simulink model "TestonBESSPVPlant"  (R2026a)
settings: Solver=VariableStepAuto  StopTime=SimulationTime  FixedStep=Ts
PreLoadFcn:
  | testModelparameters;
undefined symbols (not defined in the file): Array, Base, battery, BatteryInverter, DiscIntNeverNeededParam, fRT, GFLBatteryController, GFMBatteryController, Grid, LVRT, Panel, PVController, PVInverter, Qtrack, Ts, VSMbase
libraries: nesl_utility x16, eeGeneralControl x15, ee_lib x10, simulink x7, eeTransforms x6, fl_lib x5, eePowerMeasurement x5, slpidlib x2, batteryecm_lib x1, simulink_extras x1
(part 2 of 3)

== system TestonBESSPVPlant/BESS PV PARK/60 MWhr Battery Energy Storage/Variant Subsystem/Grid Forming VSM ==
  In Bus Element : Inport  PortName=Bat  Element=Iabc_bat
  In Bus Element1 : Inport  PortName=Bat  Element=Vabc_bat
  Constant : Constant  Value=GFMBatteryController.P_ref*0 +0.3  SampleTime=Ts
  Constant1 : Constant  Value=GFMBatteryController.Q_ref*0+0.01  SampleTime=Ts
  From Workspace : FromWorkspace  VariableName=reference.Flat  SampleTime=Ts
  From Workspace1 : FromWorkspace  VariableName=reference.Flat  SampleTime=Ts
  GridFormingController : Subsystem  mask(Grid-Forming Controller){power=VSMbase.power*1e3, girdLineVoltage=VSMbase.lineVoltage, powerFreq=VSMbase.frequency, dcBusVoltage=BatteryInverter.DCVoltage, measSampleTime=GFMBatteryController.Sampletime, powerControl=Virtual Synchronous Machine, activePowerSampleTime=GFMBatteryController.Sampletime, droopSlope=BatteryInverter.droopControl.freqSlopeMp, droopT1=BatteryInverter.droopControl.T1, droopT2=BatteryInverter.droopControl.T2, droopTC=BatteryInverter.droopControl.lpfTimeConst, vsmPmeasFilterTC=GFMBatteryController.filtertimeconstant, vsmFreqDroop=1/GFMBatteryController.frequencydroop, vsmInertiaTC=GFMBatteryController.VSMInertia, vsmDampingConst=GFMBatteryController.Damping, dampingPowerMaxLimit=1, dampingPowerMinLimit=-1, freqMeasTimeConst=GFMBatteryController.frequencymeastimeconstant, freqOption=Grid Frequency Measurement, voltreference=GFMBatteryController.voltagref, QVoltFilterTC=GFMBatteryController.reactivepowerfiltertimeconstant, QVoltDroop=GFMBatteryController.voltagedroop, lowVoltageSupportGain=GFMBatteryController.voltagsupportgain, currentLimit=Virtual Impedance and Current Limiting, maxSatCurrentLimit=BatteryInverter.currentLimit.overNominalCurrent, maxVICurrentLimit=GFMBatteryController.maximumvirtualimpedancecurrent, ctLimitVirtualImp=BatteryInverter.currentLimit.virImpResistance, ctLimitXbyR=BatteryInverter.currentLimit.virImpXbyR, ctLimitDelayTime=10*GFMBatteryController.Sampletime, currentSatTime=0.001, currentVITimeConst=GFMBatteryController.virtimeconstant, modeTransferTime=0.01, voltControlTs=GFMBatteryController.voltagecontroltimeconstant, vdPGain=GFMBatteryController.voltagecontrolkp, VdIGain=GFMBatteryController.voltagecontrolki, VdMaxCt=1.8, VdMinCt=-1.8, VqPGain=GFMBatteryController.voltagecontrolkp, VqIGain=GFMBatteryController.voltagecontrolki, VqMaxCt=1.8, VqMinCt=-1.8, vdvqLPFTimeConst=GFMBatteryController.voltagecontroltimeconstant, currentControlTs=GFMBatteryController.currentcontrollersampletime, filterInductance=BatteryInverter.L, IdPGain=GFMBatteryController.currentcontrollerkp, IdIGain=GFMBatteryController.currentcontrollerki, IqPGain=GFMBatteryController.currentcontrollerkp, IqIGain=GFMBatteryController.currentcontrollerki}
      mask prompts: power "Grid-forming converter power (VA)"; girdLineVoltage "Grid line voltage (V)"; powerFreq "Grid frequency (Hz)"; dcBusVoltage "DC bus voltage (V)"; measSampleTime "Measurement sample time (s)"; powerControl "Active Power Control"; activePowerSampleTime "Power controller sample time (s)"; droopSlope "Power droop slope (pu, Hz/W)"; droopT1 "Lead-Lag numerator time constant (s)"; droopT2 "Lead-Lag denominator time constant (s)"; droopTC "Filter cut-off time constant (s)"; vsmPmeasFilterTC "Power measurement filter time constant (s)"; vsmFreqDroop "Frequency droop (pu,  W/Hz)"; vsmInertiaTC "Inertia constant M (pu)"; vsmDampingConst "Damping constant (pu/Hz)"; dampingPowerMaxLimit "Damping power maximum limit (pu)"; dampingPowerMinLimit "Damping power minimum limit (pu)"; freqMeasTimeConst "Frequency measurement time constant (s)"; freqOption "Damping power frequency option"; voltreference "Voltage reference value (pu)"; QVoltFilterTC "Power measurement filter time constant (s)"; QVoltDroop "Voltage droop (pu, V/VAr)"; lowVoltageSupportGain "Low voltage support gain (pu, A/V)"; currentLimit "Current limiting method"; maxSatCurrentLimit "Maximum current saturation (pu)"; maxVICurrentLimit "Maximum virtual impedance current (pu)"; ctLimitVirtualImp "Virtual impedance coefficient (pu.Ohm/pu.A)"; ctLimitXbyR "Virtual X/R ratio"; ctLimitDelayTime "Maximum current delay time (s)"; currentSatTime "Current limiting run time (s)"; currentVITimeConst "Filter time constant (s)"; modeTransferTime "Mode transfer time (s)"; voltControlTs "Voltage controller sample time (s)"; vdPGain "Vd proportional gain"; VdIGain "Vd integral gain"; VdMaxCt "Vd maximum current limit (A)"; VdMinCt "Vd minimum current limit (A)"; VqPGain "Vq proportional gain"; VqIGain "Vq integral gain"; VqMaxCt "Vq maximum current limit (A)"; VqMinCt "Vq minimum current limit (A)"; vdvqLPFTimeConst "Voltage measurement filter time constant (s)"; currentControlTs "Current controller sample time (s)"; filterInductance "Filter inductance (H)"; IdPGain "Id proportional gain"; IdIGain "Id integral gain"; IqPGain "Iq proportional gain"; IqIGain "Iq integral gain"
      mask help: This block implements the grid forming controller with fault ride through capability. Input to the controller are active and reactive power reference in per unit and the sensed three-phase phase current in amphere and phase voltage in volts.
      mask init:
      | powerChoice = get_param(gcb,'powerControl');
      | currentChoice = get_param(gcb,'currentLimit');
      | 
      | powerloc = [gcb, '/Power Control/ActivePowerControl']; 
      | currentloc = [gcb, '/Current Limiting/CurrentLimitingMethod'];
      | freqLoc = [gcb,'/Power Control/ActivePowerControl/vsmControl/Damping Frequency'];
      | 
      | switch powerChoice
      |     case 'Virtual Synchronous Machine'
      |         set_param(powerloc, 'LabelModeActiveChoice', 'vsm');
      |         dampingFreqChoice = get_param(gcb,'freqOption');
      |         if strcmp(dampingFreqChoice,'Grid Frequency Measurement')
      |             set_param(freqLoc, 'LabelModeActiveChoice', 'freqMeas');
      |         else
      |             set_param(freqLoc, 'LabelModeActiveChoice', 'constFreq');
      |         end
      |     case 'Droop Control'
      |          set_param(powerloc, 'LabelModeActiveChoice', 'droop');
      |    otherwise
      |         disp('Choose proper active power control method')
      | end
      | switch currentChoice
      |     case 'Virtual Impedance'
      |           set_param(currentloc, 'LabelModeActiveChoice', 'virimp');
      |     case 'Current Limiting'
      |          set_param(currentloc, 'LabelModeActiveChoice', 'ctSat');
      |     case 'Virtual Impedance and Current Limiting'
      |             set_param(currentloc, 'LabelModeActiveChoice', 'both');
      |     otherwise
      |         disp('Choose proper current limiting method')
      | end
      mask Help: This block implements the grid forming controller with fault ride through capability. Input to the controller are active and reactive power reference in per unit and the sensed three-phase phase current in amphere and phase voltage in volts.
      mask TypeOptions powerControl: Virtual Synchronous Machine | Droop Control
      mask Callback powerControl:
      | h = Simulink.Mask.get(gcb);
      | slectedActivePowerControl=get_param(gcb,'powerControl');
      | %slectedActivePowerControl = h.Parameters(find(string({h.Parameters.Name}) == 'powerControl')).Value;
      | switch slectedActivePowerControl
      |     case 'Virtual Synchronous Machine'
      |         h.Parameters(find(string({h.Parameters.Name}) == 'droopSlope')).Visible = 'off';
      |         h.Parameters(find(string({h.Parameters.Name}) == 'droopTC')).Visible = 'off';
      |         h.Parameters(find(string({h.Parameters.Name}) == 'droopT1')).Visible = 'off';
      |         h.Parameters(find(string({h.Parameters.Name}) == 'droopT2')).Visible = 'off';
      |         h.Parameters(find(string({h.Parameters.Name}) == 'vsmPmeasFilterTC')).Visible = 'on';
      |         h.Parameters(find(string({h.Parameters.Name}) == 'vsmFreqDroop')).Visible = 'on';
      |         h.Parameters(find(string({h.Parameters.Name}) == 'vsmInertiaTC')).Visible = 'on';
      |         h.Parameters(find(string({h.Parameters.Name}) == 'vsmDampingConst')).Visible = 'on';
      |         h.Parameters(find(string({h.Parameters.Name}) == 'dampingPowerMaxLimit')).Visible = 'on';
      |         h.Parameters(find(string({h.Parameters.Name}) == 'dampingPowerMinLimit')).Visible = 'on';
      |         h.Parameters(find(string({h.Parameters.Name}) == 'freqOption')).Visible = 'on';
      |         h.Parameters(find(string({h.Parameters.Name}) == 'freqMeasTimeConst')).Visible = 'on';
      |     case 'Droop Control'
      |         h.Parameters(find(string({h.Parameters.Name}) == 'droopSlope')).Visible = 'on';
      |         h.Parameters(find(string({h.Parameters.Name}) == 'droopTC')).Visible = 'on';
      |         h.Parameters(find(string({h.Parameters.Name}) == 'droopT1')).Visible = 'on';
      |         h.Parameters(find(string({h.Parameters.Name}) == 'droopT2')).Visible = 'on';
      |         h.Parameters(find(string({h.Parameters.Name}) == 'vsmPmeasFilterTC')).Visible = 'off';
      |         h.Parameters(find(string({h.Parameters.Name}) == 'vsmFreqDroop')).Visible = 'off';
      |         h.Parameters(find(string({h.Parameters.Name}) == 'vsmInertiaTC')).Visible = 'off';
      |         h.Parameters(find(string({h.Parameters.Name}) == 'vsmDampingConst')).Visible = 'off';
      |         h.Parameters(find(string({h.Parameters.Name}) == 'dampingPowerMaxLimit')).Visible = 'off';
      |         h.Parameters(find(string({h.Parameters.Name}) == 'dampingPowerMinLimit')).Visible = 'off';
      |         h.Parameters(find(string({h.Parameters.Name}) == 'freqOption')).Visible = 'off';
      |         h.Parameters(find(string({h.Parameters.Name}) == 'freqMeasTimeConst')).Visible = 'on';
      | 
      |     otherwise
      |         disp('Choose proper active power control method')
      | end
      mask TypeOptions freqOption: Grid Frequency Measurement | Constant Frequency Reference
      mask TypeOptions currentLimit: Virtual Impedance | Current Limiting | Virtual Impedance and Current Limiting
      mask Callback currentLimit:
      | h = Simulink.Mask.get(gcb);
      | currentLimitControl=get_param(gcb,'currentLimit');
      | %slectedActivePowerControl = h.Parameters(find(string({h.Parameters.Name}) == 'powerControl')).Value;
      | switch currentLimitControl
      |     case 'Virtual Impedance'
      |         h.Parameters(find(string({h.Parameters.Name}) == 'maxVICurrentLimit')).Visible = 'on';
      |         h.Parameters(find(string({h.Parameters.Name}) == 'ctLimitVirtualImp')).Visible = 'on';
      |         h.Parameters(find(string({h.Parameters.Name}) == 'ctLimitXbyR')).Visible = 'on';
      |         h.Parameters(find(string({h.Parameters.Name}) == 'maxSatCurrentLimit')).Visible = 'off';
      |         h.Parameters(find(string({h.Parameters.Name}) == 'ctLimitDelayTime')).Visible = 'off';
      |         h.Parameters(find(string({h.Parameters.Name}) == 'currentSatTime')).Visible = 'off';
      |         h.Parameters(find(string({h.Parameters.Name}) == 'currentVITimeConst')).Visible = 'on';
      |         h.Parameters(find(string({h.Parameters.Name}) == 'modeTransferTime')).Visible = 'off';
      | 
      | 
      |     case 'Current Limiting'
      |         h.Parameters(find(string({h.Parameters.Name}) == 'maxVICurrentLimit')).Visible = 'off';
      |         h.Parameters(find(string({h.Parameters.Name}) == 'ctLimitVirtualImp')).Visible = 'off';
      |         h.Parameters(find(string({h.Parameters.Name}) == 'ctLimitXbyR')).Visible = 'off';
      |         h.Parameters(find(string({h.Parameters.Name}) == 'maxSatCurrentLimit')).Visible = 'on';
      |         h.Parameters(find(string({h.Parameters.Name}) == 'ctLimitDelayTime')).Visible = 'on';
      |         h.Parameters(find(string({h.Parameters.Name}) == 'currentSatTime')).Visible = 'off';
      |         h.Parameters(find(string({h.Parameters.Name}) == 'currentVITimeConst')).Visible = 'off';
      |         h.Parameters(find(string({h.Parameters.Name}) == 'modeTransferTime')).Visible = 'off';
      | 
      |     case 'Virtual Impedance and Current Limiting'
      |         h.Parameters(find(string({h.Parameters.Name}) == 'maxVICurrentLimit')).Visible = 'on';
      |         h.Parameters(find(string({h.Parameters.Name}) == 'ctLimitVirtualImp')).Visible = 'on';
      |         h.Parameters(find(string({h.Parameters.Name}) == 'ctLimitXbyR')).Visible = 'on';
      |         h.Parameters(find(string({h.Parameters.Name}) == 'maxSatCurrentLimit')).Visible = 'on';
      |         h.Parameters(find(string({h.Parameters.Name}) == 'ctLimitDelayTime')).Visible = 'off';
      |         h.Parameters(find(string({h.Parameters.Name}) == 'currentSatTime')).Visible = 'on';
      |         h.Parameters(find(string({h.Parameters.Name}) == 'currentVITimeConst')).Visible = 'on';
      |         h.Parameters(find(string({h.Parameters.Name}) == 'modeTransferTime')).Visible = 'on';
      | 
      |     otherwise
      |         disp('Choose proper current limiting method')
      | end
      mask DialogControl ParameterGroupVar Prompt: Grid-Forming Controller Parameters
      mask DialogControl GFMGroup Prompt: Grid-Forming Converter Specifications
      mask DialogControl Pcontrolgrp Prompt: Active Power Controller Parameters
      mask DialogControl QcontrolGrp Prompt: Reactive Power Controller Parameters
      mask DialogControl faultRideThroughGrp Prompt: Fault Ride-Through Parameters
      mask DialogControl voltControlgrp Prompt: Voltage Controller Parameters
      mask DialogControl Container15currentContGrp Prompt: Current Controller Parameters
  Product : Product
  Product1 : Product
  Terminator : Terminator
  Unit Delay2 : UnitDelay  SampleTime=Ts
  mabc : Outport
  wires:
  GridFormingController/4(fmeas) -> Terminator/1  "Freq"
  In Bus Element/1 -> GridFormingController/3(Igabc)
  GridFormingController/1(mabc) -> Unit Delay2/1  "mabc"
  GridFormingController/3(Qmeas) -> [Qmeas]  "Qmeas"
  GridFormingController/2(Pmeas) -> [Pmeas]  "Pmeas"
  In Bus Element1/1 -> GridFormingController/4(Vgabc)
  Unit Delay2/1 -> mabc/1
  From Workspace/1 -> Product/1
  Constant/1 -> Product/2
  Product/1 -> GridFormingController/1(Pref)
  From Workspace1/1 -> Product1/2
  Constant1/1 -> Product1/1
  Product1/1 -> GridFormingController/2(Qref)

== system TestonBESSPVPlant/BESS PV PARK/PV Plant Controller /Voltage VAR Control & LVRT, FRT/Frequency RideThrough ==
  f : Inport
  Avoid Operation : Subsystem
  Discrete-Time Integrator1 : DiscreteIntegrator  ExternalReset=either  SampleTime=Ts  ICPrevOutput=DiscIntNeverNeededParam  ICPrevScaledInput=DiscIntNeverNeededParam
  Duration of f<fth : Lookup_n-D  NumberOfTableDimensions=1  BreakpointsForDimension1=(1+[-0.021,-0.02,0.02,0.021])*Grid.frequency  Table=[1,0,0,1]  InterpMethod=Flat  InternalRulePriority=Speed  RndMeth=Simplest
  Frequency vs Trip time : Lookup_n-D  NumberOfTableDimensions=1  BreakpointsForDimension1=fRT.frequency_x  Table=fRT.time_y  InterpMethod=Flat  InternalRulePriority=Speed  RndMeth=Simplest
  GreaterThan : RelationalOperator  Operator=>  OutDataTypeStr=boolean  RndMeth=Simplest  InputSameDT=off
  Trip  Signal : Outport
  wires:
  Discrete-Time Integrator1/1 -> GreaterThan/1
  Frequency vs Trip time/1 -> GreaterThan/2
  GreaterThan/1 -> Trip  Signal/1
  Duration of f<fth/1 -> Discrete-Time Integrator1/2, Discrete-Time Integrator1/1
  Avoid Operation/1(f) -> Duration of f<fth/1, Frequency vs Trip time/1
  f/1 -> Avoid Operation/1(f_in)

== system TestonBESSPVPlant/BESS PV PARK/PV Plant Controller /Voltage VAR Control & LVRT, FRT/LVRT Characterstics ==
  Vmag : Inport
  Discrete-Time Integrator1 : DiscreteIntegrator  ExternalReset=either  SampleTime=Ts  ICPrevOutput=DiscIntNeverNeededParam  ICPrevScaledInput=DiscIntNeverNeededParam
  Duration of Vmag<Vth : Lookup_n-D  NumberOfTableDimensions=1  BreakpointsForDimension1=[0,.9,0.91,1.2]  Table=[1,1,0,0]  InterpMethod=Flat  InternalRulePriority=Speed  RndMeth=Simplest
  Gain1 : Gain  Gain=-1
  GreaterThan : RelationalOperator  Operator=>  OutDataTypeStr=boolean  RndMeth=Simplest  InputSameDT=off
  Saturation2 : Saturate  UpperLimit=1  LowerLimit=-1
  Vmag vs Trip time : Lookup_n-D  NumberOfTableDimensions=1  BreakpointsForDimension1=LVRT.voltage_x  Table=LVRT.time_y  InterpMethod=Flat  InternalRulePriority=Speed  RndMeth=Simplest
  Vmag vs iq : Lookup_n-D  NumberOfTableDimensions=1  BreakpointsForDimension1=LVRT.volatge_iq_x  Table=LVRT.iq_y  InternalRulePriority=Speed  RndMeth=Simplest
  Trip Signal : Outport
  iq : Outport  Port=2
  wires:
  Duration of Vmag<Vth/1 -> Discrete-Time Integrator1/2, Discrete-Time Integrator1/1
  GreaterThan/1 -> Trip Signal/1
  Discrete-Time Integrator1/1 -> GreaterThan/1
  Vmag vs Trip time/1 -> GreaterThan/2
  Vmag vs iq/1 -> Saturation2/1
  Gain1/1 -> iq/1
  Saturation2/1 -> Gain1/1
  Vmag/1 -> Vmag vs iq/1, Vmag vs Trip time/1, Duration of Vmag<Vth/1

== system TestonBESSPVPlant/BESS PV PARK/PV Plant Controller /Voltage VAR Control & LVRT, FRT/Voltage Control ==
  In1 : Inport
  In2 : Inport  Port=2
  Constant2 : Constant  Value=0
  Gain : Gain  Gain=PVController.m_v
  Sum2 : Sum  Inputs=|+-
  Switch1 : Switch  Threshold=.9  SaturateOnIntegerOverflow=off  InputSameDT=off
  Out1 : Outport
  wires:
  Gain/1 -> Out1/1
  Sum2/1 -> Switch1/1
  Switch1/1 -> Gain/1
  In1/1 -> Sum2/2, Switch1/2
  Constant2/1 -> Switch1/3
  In2/1 -> Sum2/1

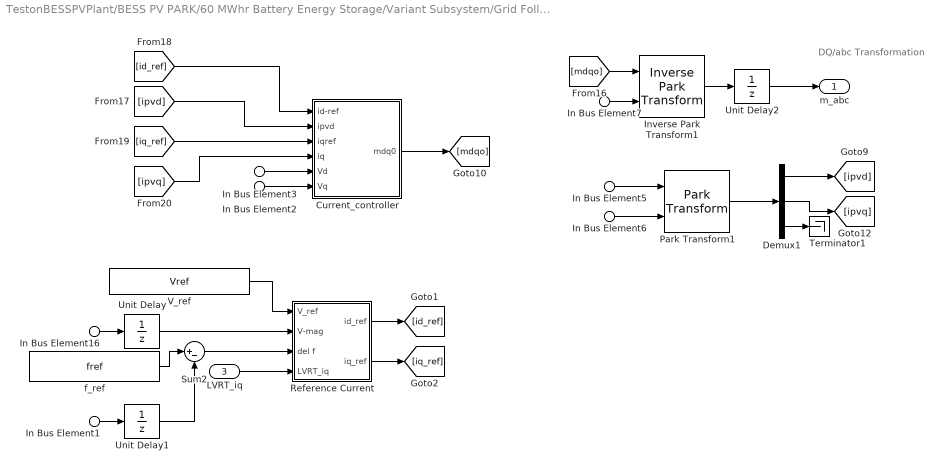
== system TestonBESSPVPlant/BESS PV PARK/60 MWhr Battery Energy Storage/Variant Subsystem/Grid Following Support/GFL Battery Controller ==
  note: DQ/abc Transformation
  In Bus Element3 : Inport  PortName=Vbus  Element=Vd
  In Bus Element16 : Inport  PortName=Vbus  Element=Vd
  In Bus Element2 : Inport  PortName=Vbus  Element=Vq
  In Bus Element6 : Inport  PortName=Vbus  Element=Theta
  In Bus Element7 : Inport  PortName=Vbus  Element=Theta
  In Bus Element1 : Inport  PortName=Vbus  Element=w
  In Bus Element5 : Inport  Port=2  PortName=ipv2  Element=1
  LVRT_iq : Inport  Port=3
  Current_controller : Subsystem
  Demux1 : Demux  Outputs=3
  Inverse Park Transform1 : eeTransforms/Inverse Park Transform  AxisAlignment=Q-axis  PowerInvariant=off
  Park Transform1 : eeTransforms/Park Transform  AxisAlignment=Q-axis  PowerInvariant=off
  Reference Current : Subsystem
  Sum2 : Sum  Inputs=|+-
  Terminator1 : Terminator
  Unit Delay : UnitDelay  SampleTime=Td
  Unit Delay1 : UnitDelay  SampleTime=Td
  Unit Delay2 : UnitDelay  SampleTime=Ts
  V_ref : Constant  Value=Vref
  f_ref : Constant  Value=fref
  m_abc : Outport
  wires:
  In Bus Element2/1 -> Current_controller/6(Vq)
  Current_controller/1(mdq0) -> [mdqo]
  Inverse Park Transform1/1 -> Unit Delay2/1
  Demux1/2 -> [ipvq]
  Unit Delay2/1 -> m_abc/1
  Demux1/1 -> [ipvd]
  Demux1/3 -> Terminator1/1
  [mdqo] -> Inverse Park Transform1/1
  Park Transform1/1 -> Demux1/1
  [id_ref] -> Current_controller/1(id-ref)
  In Bus Element3/1 -> Current_controller/5(Vd)
  [iq_ref] -> Current_controller/3(iqref)
  [ipvq] -> Current_controller/4(iq)
  In Bus Element6/1 -> Park Transform1/2
  In Bus Element7/1 -> Inverse Park Transform1/2
  [ipvd] -> Current_controller/2(ipvd)
  In Bus Element5/1 -> Park Transform1/1
  f_ref/1 -> Sum2/1
  V_ref/1 -> Reference Current/1(V_ref)
  In Bus Element16/1 -> Unit Delay/1
  LVRT_iq/1 -> Reference Current/4(LVRT_iq)
  Sum2/1 -> Reference Current/3(del f)
  Reference Current/2(iq_ref) -> [iq_ref]
  Reference Current/1(id_ref) -> [id_ref]
  In Bus Element1/1 -> Unit Delay1/1
  Unit Delay1/1 -> Sum2/2
  Unit Delay/1 -> Reference Current/2(V-mag)

== system TestonBESSPVPlant/BESS PV PARK/60 MWhr Battery Energy Storage/Variant Subsystem/Grid Forming VSM/GridFormingController ==
  Pref : Inport
  Qref : Inport  Port=2
  Igabc : Inport  Port=3
  Vgabc : Inport  Port=4
  Current Limiting : Subsystem
  Grid Voltage Reactive Power Support : Subsystem
  Measurement : Subsystem
      mask Display: image('meas2_1.png');
  Power Control : Subsystem
  VoltageCurrentControl : Subsystem
      settings: PortSchema="{\"entries\":[{\"content\":{\"sides\":[{\"content\":{\"connectorIds\":[\"In1\",\"In2\"]},\"type\":\"ConnectorPlacement.EquallySpacedRectSide\",\"uuid\":\"0bf15a12-7bc0-47e4-89bd-435769673763\"},{\"content\":{\"connectorIds\":[\"Out1\"],\"side\":\"RIGHT\"},\"type\":\"ConnectorPlacement.EquallySpacedRectSide\",\"uuid\":\"44a15d74-8878-4ec6-abe4-be0b1b609519\"},{\"content\":{\"connectorIds\":[\"In3\"],\"side\":\"TOP\"},\"type\":\"ConnectorPlacement.EquallySpacedRectSide\",\"uuid\":\"7a96781e-5638-4b2a-8101-d5785aae9f0f\"}]},\"type\":\"ConnectorPlacement.EquallySpacedConnector\",\"uuid\":\"4b3373ad-cf20-4175-894e-3bd1604dd0ce\"}],\"packageUris\":[\"http://schema.mathworks.com/mf0/Connector/R2020b\"],\"version\":\"1.0\"}"
  mabc : Outport
  Pmeas : Outport  Port=2
  Qmeas : Outport  Port=3
  fmeas : Outport  Port=4
  wires:
  VoltageCurrentControl/1(mabc) -> mabc/1
  Vgabc/1 -> Measurement/1(Vgabcc)
  Igabc/1 -> Measurement/2(Igabc)
  Measurement/2(Pmeas) -> Pmeas/1
  Measurement/3(Qmeas) -> Qmeas/1
  Measurement/1(measure) -> Current Limiting/1(measure), VoltageCurrentControl/3(measure), Power Control/1(measure), Grid Voltage Reactive Power Support/1(measure)
  Power Control/3(angle) -> Measurement/3(Angle)
  Power Control/1(reactiveControl) -> Current Limiting/2(reactiveControl)
  Power Control/2(activeControl) -> VoltageCurrentControl/2(activeControl)
  Current Limiting/1(currentLimiting) -> VoltageCurrentControl/1(currentLimiting)
  Qref/1 -> Grid Voltage Reactive Power Support/3(QrefInput)
  Pref/1 -> Grid Voltage Reactive Power Support/2(PrefInput)
  Grid Voltage Reactive Power Support/1(Pref) -> Power Control/2(Pref)
  Grid Voltage Reactive Power Support/2(Qref) -> Power Control/3(Qref)
  Measurement/4(fmeas) -> fmeas/1

== system TestonBESSPVPlant/BESS PV PARK/PV Plant Controller /Voltage VAR Control & LVRT, FRT/Frequency RideThrough/Avoid Operation ==
  f_in : Inport
  Constant : Constant  Value=Grid.frequency  SampleTime=Ts
  Step : Step  Time=0.5  SampleTime=Ts
  Switch : Switch  Criteria=u2 > Threshold  SaturateOnIntegerOverflow=off  InputSameDT=off
  f : Outport
  wires:
  f_in/1 -> Switch/1
  Constant/1 -> Switch/3
  Step/1 -> Switch/2
  Switch/1 -> f/1

== system TestonBESSPVPlant/BESS PV PARK/60 MWhr Battery Energy Storage/Variant Subsystem/Grid Following Support/GFL Battery Controller/Current_controller ==
  id-ref : Inport
  ipvd : Inport  Port=2
  iqref : Inport  Port=3
  iq : Inport  Port=4
  Vd : Inport  Port=5
  Vq : Inport  Port=6
  Constant4 : Constant  Value=0
  Gain1 : Gain  Gain=2*1*pi*60*L/zbase
  Gain2 : Gain  Gain=2*1*pi*60*L/zbase
  Mux1 : Mux  Inputs=3
  PID Controller : slpidlib/PID Controller  Controller=PID  Form=Parallel  TimeDomain=Discrete-time  UseExternalTs=off  SampleTime=-1  IntegratorMethod=Forward Euler  FilterMethod=Forward Euler  ControllerParametersSource=internal  P=Kpic  I=Kiic  UseKiTs=off  D=Kd  UseExternalDerivativeSource=off  N=100  UseFilter=on  TunerSelectOption=Transfer Function Based (PID Tuner App)  InitialConditionSource=internal  InitialConditionForIntegrator=0  InitialConditionForFilter=0  DifferentiatorICPrevScaledInput=0  ExternalReset=none  TrackingMode=off  Kt=1  LimitOutput=off  SatLimitsSource=internal  UpperSaturationLimit=inf  LowerSaturationLimit=-inf  LinearizeAsGain=on  AntiWindupMode=none  Kb=1  LimitIntegrator=off  UpperIntegratorSaturationLimit=inf  LowerIntegratorSaturationLimit=-inf  POutMin=[]  POutMax=[]  IOutMin=[]  IOutMax=[]  DOutMin=[]  DOutMax=[]  NOutMin=[]  NOutMax=[]  SumOutMin=[]  SumOutMax=[]  SaturationOutMin=[]  SaturationOutMax=[]  PParamMin=[]  PParamMax=[]  IParamMin=[]  IParamMax=[]  DParamMin=[]  DParamMax=[]  NParamMin=[]  NParamMax=[]  KbParamMin=[]  KbParamMax=[]  KtParamMin=[]  KtParamMax=[]  KbOutMin=[]  KbOutMax=[]  KtOutMin=[]  KtOutMax=[]  IntegratorOutMin=[]  IntegratorOutMax=[]  FilterOutMin=[]  FilterOutMax=[]  SumI1OutMin=[]  SumI1OutMax=[]  SumI2OutMin=[]  SumI2OutMax=[]  SumI3OutMin=[]  SumI3OutMax=[]  SumI4OutMin=[]  SumI4OutMax=[]  SumDOutMin=[]  SumDOutMax=[]  DifferentiatorOutMin=[]  DifferentiatorOutMax=[]  FilterDiffOutCoefMin=[]  FilterDiffOutCoefMax=[]  ReciprocalOutMin=[]  ReciprocalOutMax=[]  SumDenOutMin=[]  SumDenOutMax=[]  SumNumOutMin=[]  SumNumOutMax=[]  DivideOutMin=[]  DivideOutMax=[]  UdiffTsProdOutMin=[]  UdiffTsProdOutMax=[]  NTsProdOutMin=[]  NTsProdOutMax=[]  UintegralTsProdOutMin=[]  UintegralTsProdOutMax=[]  UngainTsProdOutMin=[]  UngainTsProdOutMax=[]  ClampingZeroOutDataTypeStr=Inherit: Inherit via back propagation  ClampingZeroOutMin=[]  ClampingZeroOutMax=[]  FilterDenConstantOutDataTypeStr=Inherit: Inherit via back propagation  FilterDenConstantOutMin=[]  FilterDenConstantOutMax=[]  PCopyOutDataTypeStr=Inherit: Inherit via back propagation  PCopyOutMin=[]  PCopyOutMax=[]  NCopyOutDataTypeStr=Inherit: Inherit via back propagation  NCopyOutMin=[]  NCopyOutMax=[]  IntegratorContinuousStateAttributes=''  IntegratorStateMustResolveToSignalObject=off  IntegratorRTWStateStorageClass=Auto  FilterContinuousStateAttributes=''  FilterStateMustResolveToSignalObject=off  FilterRTWStateStorageClass=Auto  ParallelPVariant=InternalParameters  IdealPVariant=Disabled  IVariant=InternalParameters  DVariant=InternalParameters  IntegratorVariant=Discrete  SatVariant=Disabled  AWVariant=Passthrough  PCopyVariant=Disabled  TRVariant=Disabled  FdbkBlocksVariant=Forward  IdealPFdbkVariant=Disabled  SatFdbkVariant=Disabled  DerivativeFilterVariant=ForwardEulerFilter  NVariant=InternalParameters  NCopyVariant=Disabled  FilterICVariant=InternalICsFilter  IntegratorICVariant=InternalICs  ExternalResetVariant=Disabled  TRSumVariant=Passthrough  SumFdbkVariant=Disabled  SumVariant=Sum_PID  TsampFilterVariant=InternalTs  TsampNgainVariant=Passthrough  TsampIntegralVariant=Disabled_SignalSpec  ExternalSaturationOutDataTypeStr=Inherit: Same as second input  DerivativeSourceVariant=ErrorSignal  PreIntVariant=InternalPreInt
  PID Controller1 : slpidlib/PID Controller  Controller=PID  Form=Parallel  TimeDomain=Discrete-time  UseExternalTs=off  SampleTime=-1  IntegratorMethod=Forward Euler  FilterMethod=Forward Euler  ControllerParametersSource=internal  P=Kpic  I=Kiic  UseKiTs=off  D=Kd  UseExternalDerivativeSource=off  N=100  UseFilter=on  TunerSelectOption=Transfer Function Based (PID Tuner App)  InitialConditionSource=internal  InitialConditionForIntegrator=0  InitialConditionForFilter=0  DifferentiatorICPrevScaledInput=0  ExternalReset=none  TrackingMode=off  Kt=1  LimitOutput=off  SatLimitsSource=internal  UpperSaturationLimit=inf  LowerSaturationLimit=-inf  LinearizeAsGain=on  AntiWindupMode=none  Kb=1  LimitIntegrator=off  UpperIntegratorSaturationLimit=inf  LowerIntegratorSaturationLimit=-inf  POutMin=[]  POutMax=[]  IOutMin=[]  IOutMax=[]  DOutMin=[]  DOutMax=[]  NOutMin=[]  NOutMax=[]  SumOutMin=[]  SumOutMax=[]  SaturationOutMin=[]  SaturationOutMax=[]  PParamMin=[]  PParamMax=[]  IParamMin=[]  IParamMax=[]  DParamMin=[]  DParamMax=[]  NParamMin=[]  NParamMax=[]  KbParamMin=[]  KbParamMax=[]  KtParamMin=[]  KtParamMax=[]  KbOutMin=[]  KbOutMax=[]  KtOutMin=[]  KtOutMax=[]  IntegratorOutMin=[]  IntegratorOutMax=[]  FilterOutMin=[]  FilterOutMax=[]  SumI1OutMin=[]  SumI1OutMax=[]  SumI2OutMin=[]  SumI2OutMax=[]  SumI3OutMin=[]  SumI3OutMax=[]  SumI4OutMin=[]  SumI4OutMax=[]  SumDOutMin=[]  SumDOutMax=[]  DifferentiatorOutMin=[]  DifferentiatorOutMax=[]  FilterDiffOutCoefMin=[]  FilterDiffOutCoefMax=[]  ReciprocalOutMin=[]  ReciprocalOutMax=[]  SumDenOutMin=[]  SumDenOutMax=[]  SumNumOutMin=[]  SumNumOutMax=[]  DivideOutMin=[]  DivideOutMax=[]  UdiffTsProdOutMin=[]  UdiffTsProdOutMax=[]  NTsProdOutMin=[]  NTsProdOutMax=[]  UintegralTsProdOutMin=[]  UintegralTsProdOutMax=[]  UngainTsProdOutMin=[]  UngainTsProdOutMax=[]  ClampingZeroOutDataTypeStr=Inherit: Inherit via back propagation  ClampingZeroOutMin=[]  ClampingZeroOutMax=[]  FilterDenConstantOutDataTypeStr=Inherit: Inherit via back propagation  FilterDenConstantOutMin=[]  FilterDenConstantOutMax=[]  PCopyOutDataTypeStr=Inherit: Inherit via back propagation  PCopyOutMin=[]  PCopyOutMax=[]  NCopyOutDataTypeStr=Inherit: Inherit via back propagation  NCopyOutMin=[]  NCopyOutMax=[]  IntegratorContinuousStateAttributes=''  IntegratorStateMustResolveToSignalObject=off  IntegratorRTWStateStorageClass=Auto  FilterContinuousStateAttributes=''  FilterStateMustResolveToSignalObject=off  FilterRTWStateStorageClass=Auto  ParallelPVariant=InternalParameters  IdealPVariant=Disabled  IVariant=InternalParameters  DVariant=InternalParameters  IntegratorVariant=Discrete  SatVariant=Disabled  AWVariant=Passthrough  PCopyVariant=Disabled  TRVariant=Disabled  FdbkBlocksVariant=Forward  IdealPFdbkVariant=Disabled  SatFdbkVariant=Disabled  DerivativeFilterVariant=ForwardEulerFilter  NVariant=InternalParameters  NCopyVariant=Disabled  FilterICVariant=InternalICsFilter  IntegratorICVariant=InternalICs  ExternalResetVariant=Disabled  TRSumVariant=Passthrough  SumFdbkVariant=Disabled  SumVariant=Sum_PID  TsampFilterVariant=InternalTs  TsampNgainVariant=Passthrough  TsampIntegralVariant=Disabled_SignalSpec  ExternalSaturationOutDataTypeStr=Inherit: Same as second input  DerivativeSourceVariant=ErrorSignal  PreIntVariant=InternalPreInt
  Sum1 : Sum  Inputs=|+-
  Sum3 : Sum  Inputs=|++-
  Sum4 : Sum  Inputs=|+++
  Sum5 : Sum  Inputs=|+-
  mdq0 : Outport
  wires:
  PID Controller/1 -> Sum3/2
  Sum3/1 -> Mux1/1, [Ed]
  Gain2/1 -> Sum3/3
  ipvd/1 -> Gain1/1, Sum1/2
  id-ref/1 -> Sum1/1
  Gain1/1 -> Sum4/3
  Vq/1 -> Sum4/2
  iq/1 -> Gain2/1, Sum5/2
  Sum1/1 -> PID Controller/1
  Vd/1 -> Sum3/1
  Constant4/1 -> Mux1/3
  Sum5/1 -> PID Controller1/1
  iqref/1 -> Sum5/1
  PID Controller1/1 -> Sum4/1
  Sum4/1 -> Mux1/2, [Eq]
  Mux1/1 -> mdq0/1

== system TestonBESSPVPlant/BESS PV PARK/60 MWhr Battery Energy Storage/Variant Subsystem/Grid Following Support/GFL Battery Controller/Reference Current ==
  note: Refernce Generation
  note: Current Limiters
  note: Avoid division by zero during start
  V_ref : Inport
  V-mag : Inport  Port=2
  del f : Inport  Port=3
  LVRT_iq : Inport  Port=4
  Constant : Constant  Value=Qref
  Constant1 : Constant
  Constant3 : Constant  Value=Imax
  Current limits : Subsystem
  Refernce id generation : Subsystem
  Refernce iq generation : Subsystem
  Switch : Switch  Criteria=u2 ~= 0  SaturateOnIntegerOverflow=off  InputSameDT=off
  Unit Delay1 : UnitDelay  SampleTime=Ts
  Unit Delay3 : UnitDelay  SampleTime=Ts
  id_ref : Outport
  iq_ref : Outport  Port=2
  wires:
  Current limits/1(iubd) -> [ubid]
  Unit Delay1/1 -> Current limits/2(iqref)
  Current limits/2(iubq) -> [ubiq]
  Unit Delay3/1 -> Current limits/3(idref)
  Constant3/1 -> Current limits/1(Imax)
  Refernce id generation/1(id_ref) -> id_ref/1, Unit Delay3/1
  del f/1 -> Refernce id generation/2(del f)
  V_ref/1 -> Refernce iq generation/1(V_ref)
  Refernce iq generation/1(iq_ref) -> Unit Delay1/1, iq_ref/1
  LVRT_iq/1 -> Refernce iq generation/3(LVRT_iq)
  [ubiq] -> Refernce iq generation/4(ubiq)
  [ubid] -> Refernce id generation/3(ubid)
  V-mag/1 -> Switch/1, Switch/2
  Switch/1 -> Refernce id generation/1(V_mag), Refernce iq generation/2(V_mag)
  Constant1/1 -> Switch/3
  Constant/1 -> Refernce iq generation/5(Q_ref)

== system TestonBESSPVPlant/BESS PV PARK/60 MWhr Battery Energy Storage/Variant Subsystem/Grid Forming VSM/GridFormingController/Current Limiting ==
  In Bus Element : Inport  PortName=measure  Element=Igd
  In Bus Element1 : Inport  PortName=measure  Element=Igq
  In Bus Element2 : Inport  Port=2  PortName=reactiveControl  Element=Vmd
  In Bus Element4 : Inport  Port=2  PortName=reactiveControl  Element=Vmq
  CurrentLimitingMethod : Subsystem  Variant=on  VariantControlMode=label  VariantControl=Choice  LabelModeActiveChoice=both
  Subtract : Sum  Inputs=+-
  Subtract1 : Sum  Inputs=-+
  Out Bus Element : Outport  PortName=currentLimiting  Element=Vmd
  Out Bus Element1 : Outport  PortName=currentLimiting  Element=Vmq
  Out Bus Element2 : Outport  PortName=currentLimiting  Element=Idmax
  Out Bus Element3 : Outport  PortName=currentLimiting  Element=Iqmax
  wires:
  In Bus Element2/1 -> Subtract/1
  In Bus Element1/1 -> CurrentLimitingMethod/2(Igq)
  In Bus Element4/1 -> Subtract1/2
  Subtract/1 -> Out Bus Element/1
  Subtract1/1 -> Out Bus Element1/1
  CurrentLimitingMethod/4(Iqmax) -> Out Bus Element3/1
  In Bus Element/1 -> CurrentLimitingMethod/1(Igd)  "Q"
  CurrentLimitingMethod/3(Idmax) -> Out Bus Element2/1
  CurrentLimitingMethod/1(delVd) -> Subtract/2
  CurrentLimitingMethod/2(delVq) -> Subtract1/1

== system TestonBESSPVPlant/BESS PV PARK/60 MWhr Battery Energy Storage/Variant Subsystem/Grid Forming VSM/GridFormingController/Grid Voltage Reactive Power Support ==
  In Bus Element1 : Inport  PortName=measure  Element=Vgd
  In Bus Element3 : Inport  PortName=measure  Element=Vgq
  In Bus Element2 : Inport  PortName=measure  Element=Igd
  In Bus Element4 : Inport  PortName=measure  Element=Igq
  PrefInput : Inport  Port=2
  QrefInput : Inport  Port=3
  Modifying Active Power Reference : Subsystem
  Modifying Reactive Power Reference : Subsystem
  Rate Transition{1..4} (4 alike) : RateTransition
  Pref : Outport
  Qref : Outport  Port=2
  wires:
  Modifying Active Power Reference/1(Pref) -> Rate Transition3/1
  PrefInput/1 -> Modifying Active Power Reference/1(PrefInput)
  In Bus Element2/1 -> Modifying Active Power Reference/3(Igd)
  In Bus Element4/1 -> Modifying Active Power Reference/4(Igq)
  In Bus Element1/1 -> Rate Transition1/1, Modifying Active Power Reference/2(Vd)
  In Bus Element3/1 -> Rate Transition2/1
  QrefInput/1 -> Rate Transition4/1
  Modifying Reactive Power Reference/1(PrefNew) -> Pref/1
  Modifying Reactive Power Reference/2(QrefNew) -> Qref/1
  Rate Transition1/1 -> Modifying Reactive Power Reference/1(Vgd)
  Rate Transition2/1 -> Modifying Reactive Power Reference/2(Vgq)
  Rate Transition3/1 -> Modifying Reactive Power Reference/4(Pref)
  Rate Transition4/1 -> Modifying Reactive Power Reference/3(Qref)

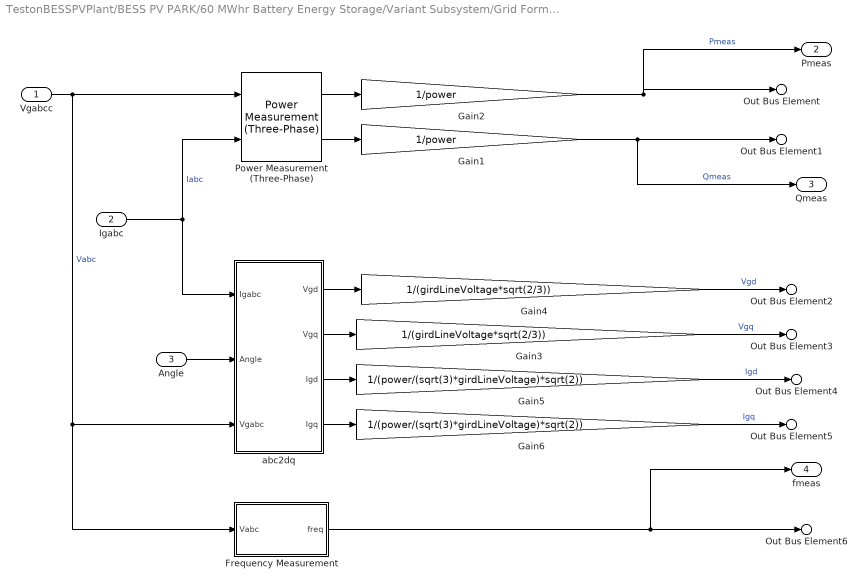
== system TestonBESSPVPlant/BESS PV PARK/60 MWhr Battery Energy Storage/Variant Subsystem/Grid Forming VSM/GridFormingController/Measurement ==
  Vgabcc : Inport
  Igabc : Inport  Port=2
  Angle : Inport  Port=3
  Frequency Measurement : Subsystem
  Gain1 : Gain  Gain=1/power
  Gain2 : Gain  Gain=1/power
  Gain3 : Gain  Gain=1/(girdLineVoltage*sqrt(2/3))
  Gain4 : Gain  Gain=1/(girdLineVoltage*sqrt(2/3))
  Gain5 : Gain  Gain=1/(power/(sqrt(3)*girdLineVoltage)*sqrt(2))
  Gain6 : Gain  Gain=1/(power/(sqrt(3)*girdLineVoltage)*sqrt(2))
  Power Measurement (Three-Phase) : eePowerMeasurement/Power Measurement (Three-Phase)  LabelModeActiveChoice=Discrete  F=powerFreq  K=[1]  Seq=Positive  Ts=measSampleTime
  abc2dq : Subsystem
  Out Bus Element : Outport  PortName=measure  Element=P
  Out Bus Element1 : Outport  PortName=measure  Element=Q
  Out Bus Element2 : Outport  PortName=measure  Element=Vgd
  Out Bus Element3 : Outport  PortName=measure  Element=Vgq
  Out Bus Element4 : Outport  PortName=measure  Element=Igd
  Out Bus Element5 : Outport  PortName=measure  Element=Igq
  Out Bus Element6 : Outport  PortName=measure  Element=fgrid
  Pmeas : Outport  Port=2
  Qmeas : Outport  Port=3
  fmeas : Outport  Port=4
  wires:
  Vgabcc/1 -> abc2dq/3(Vgabc), Frequency Measurement/1(Vabc), Power Measurement (Three-Phase)/1  "Vabc"
  Angle/1 -> abc2dq/2(Angle)
  Power Measurement (Three-Phase)/1 -> Gain2/1
  Igabc/1 -> abc2dq/1(Igabc), Power Measurement (Three-Phase)/2  "Iabc"
  Power Measurement (Three-Phase)/2 -> Gain1/1
  Gain2/1 -> Pmeas/1, Out Bus Element/1  "Pmeas"
  Gain1/1 -> Qmeas/1, Out Bus Element1/1  "Qmeas"
  abc2dq/1(Vgd) -> Gain4/1
  abc2dq/2(Vgq) -> Gain3/1
  abc2dq/3(Igd) -> Gain5/1
  abc2dq/4(Igq) -> Gain6/1
  Gain3/1 -> Out Bus Element3/1  "Vgq"
  Gain4/1 -> Out Bus Element2/1  "Vgd"
  Gain5/1 -> Out Bus Element4/1  "Igd"
  Gain6/1 -> Out Bus Element5/1  "Igq"
  Frequency Measurement/1(freq) -> Out Bus Element6/1, fmeas/1

== system TestonBESSPVPlant/BESS PV PARK/60 MWhr Battery Energy Storage/Variant Subsystem/Grid Forming VSM/GridFormingController/Power Control ==
  note: Reactive Power Control
  note: Active Power Control
  In Bus Element2 : Inport  PortName=measure  Element=P
  In Bus Element3 : Inport  PortName=measure  Element=Q
  In Bus Element1 : Inport  PortName=measure  Element=fgrid
  Pref : Inport  Port=2
  Qref : Inport  Port=3
  ActivePowerControl : Subsystem  Variant=on  VariantControlMode=label  VariantControl=Choice  LabelModeActiveChoice=vsm
  ReactiveControl : Subsystem
  Out Bus Element : Outport  PortName=reactiveControl  Element=Vmd
  Out Bus Element1 : Outport  PortName=reactiveControl  Element=Vmq
  Out Bus Element6 : Outport  Port=2  PortName=activeControl  Element=angle
  Out Bus Element4 : Outport  Port=2  PortName=activeControl  Element=w
  angle : Outport  Port=3
  wires:
  ActivePowerControl/2(w) -> Out Bus Element4/1
  In Bus Element3/1 -> ReactiveControl/2(Qmeas)
  ActivePowerControl/1(Theta) -> angle/1, Out Bus Element6/1
  ReactiveControl/1(Vmd) -> Out Bus Element/1
  ReactiveControl/2(Vmq) -> Out Bus Element1/1
  Pref/1 -> ActivePowerControl/1(Pref)  "Q"
  Qref/1 -> ReactiveControl/1(Qref)  "Q"
  In Bus Element2/1 -> ActivePowerControl/2(Pmeas)
  In Bus Element1/1 -> ActivePowerControl/3(fgrid)

== system TestonBESSPVPlant/BESS PV PARK/60 MWhr Battery Energy Storage/Variant Subsystem/Grid Forming VSM/GridFormingController/VoltageCurrentControl ==
  In Bus Element : Inport  PortName=currentLimiting  Element=Vmd
  In Bus Element1 : Inport  PortName=currentLimiting  Element=Vmq
  In Bus Element6 : Inport  PortName=currentLimiting  Element=Idmax
  In Bus Element7 : Inport  PortName=currentLimiting  Element=Iqmax
  Bus Element In6 : Inport  Port=2  PortName=activeControl  Element=w
  Bus Element In1 : Inport  Port=2  PortName=activeControl  Element=angle
  In Bus Element2 : Inport  Port=3  PortName=measure  Element=Vgd
  In Bus Element3 : Inport  Port=3  PortName=measure  Element=Vgq
  In Bus Element4 : Inport  Port=3  PortName=measure  Element=Igd
  In Bus Element5 : Inport  Port=3  PortName=measure  Element=Igq
  Controller : Subsystem
  Modulation Signal : Subsystem
  mabc : Outport
  wires:
  Controller/2(Vq) -> Modulation Signal/2(Vq)
  Modulation Signal/1(mabc) -> mabc/1
  Controller/1(Vd) -> Modulation Signal/1(Vd)
  In Bus Element4/1 -> Controller/6(Id)
  In Bus Element5/1 -> Controller/7(Iq)
  In Bus Element6/1 -> Controller/8(Idmax)
  In Bus Element7/1 -> Controller/9(Iqmax)
  In Bus Element2/1 -> Controller/4(Vsd)
  In Bus Element3/1 -> Controller/5(Vsq)
  Bus Element In6/1 -> Controller/1(Angfreq)
  In Bus Element/1 -> Controller/2(Vgdref)
  In Bus Element1/1 -> Controller/3(Vgqref)
  Bus Element In1/1 -> Modulation Signal/3(Angle)

== system TestonBESSPVPlant/BESS PV PARK/60 MWhr Battery Energy Storage/Variant Subsystem/Grid Following Support/GFL Battery Controller/Reference Current/Current limits ==
  Imax : Inport
  iqref : Inport  Port=2
  idref : Inport  Port=3
  Constant8 : Constant  Value=0
  Constant9 : Constant  Value=0
  Sqrt : Sqrt
  Sqrt1 : Sqrt
  Square{1..4} (4 alike) : Math  Operator=square
  Step2 : Step  Time=0.01  SampleTime=Ts
  Step3 : Step  Time=0.01  SampleTime=Ts
  Sum6 : Sum  Inputs=|+-
  Sum9 : Sum  Inputs=|+-
  Switch1 : Switch  Threshold=.01  SaturateOnIntegerOverflow=off  InputSameDT=off
  Switch2 : Switch  Threshold=.01  SaturateOnIntegerOverflow=off  InputSameDT=off
  iubd : Outport
  iubq : Outport  Port=2
  wires:
  Sum9/1 -> Switch2/1
  Step3/1 -> Switch2/2
  Step2/1 -> Switch1/2
  Switch2/1 -> Sqrt1/1
  Square1/1 -> Sum6/1
  Switch1/1 -> Sqrt/1
  iqref/1 -> Square2/1
  Square3/1 -> Sum9/1
  Sum6/1 -> Switch1/1
  Square2/1 -> Sum6/2
  Constant8/1 -> Switch1/3
  Square4/1 -> Sum9/2
  Constant9/1 -> Switch2/3
  Sqrt/1 -> iubd/1
  Imax/1 -> Square3/1, Square1/1
  Sqrt1/1 -> iubq/1
  idref/1 -> Square4/1

== system TestonBESSPVPlant/BESS PV PARK/60 MWhr Battery Energy Storage/Variant Subsystem/Grid Following Support/GFL Battery Controller/Reference Current/Refernce id generation ==
  V_mag : Inport
  del f : Inport  Port=2
  ubid : Inport  Port=3
  Divide : Product  Inputs=/*
  Gain6 : Gain  Gain=-1
  P/Q Priority : Switch  Criteria=u2 ~= 0  SaturateOnIntegerOverflow=off  InputSameDT=off
  PU : Gain  Gain=1/(1*Base.MVA_base_new)
  P_ref : Constant  Value=Pref
  Priority Mode : Constant  Value=P-2
  Saturation Dynamic2 : simulink/Discontinuities/Saturation Dynamic  OutMin=[]  OutMax=[]  OutDataTypeStr=Inherit: Same as second input  OutDataType=fixdt(1, 16)  OutScaling=2^-10  DoSatur=off
  Saturation1 : Saturate  UpperLimit=Imax  LowerLimit=-Imax
  Sum : Sum  Inputs=|++
  droop m_p : Gain  Gain=mp/MVA
  ubid1 : InportShadow  Port=3
  id_ref : Outport
  wires:
  P_ref/1 -> PU/1
  droop m_p/1 -> Sum/1
  Sum/1 -> Divide/2
  ubid/1 -> Saturation Dynamic2/1
  Gain6/1 -> Saturation Dynamic2/3
  Saturation Dynamic2/1 -> P/Q Priority/3
  PU/1 -> Sum/2
  Priority Mode/1 -> P/Q Priority/2
  Saturation1/1 -> P/Q Priority/1
  ubid1/1 -> Gain6/1
  P/Q Priority/1 -> id_ref/1
  V_mag/1 -> Divide/1
  Divide/1 -> Saturation1/1, Saturation Dynamic2/2
  del f/1 -> droop m_p/1

== system TestonBESSPVPlant/BESS PV PARK/60 MWhr Battery Energy Storage/Variant Subsystem/Grid Following Support/GFL Battery Controller/Reference Current/Refernce iq generation ==
  V_ref : Inport
  V_mag : Inport  Port=2
  LVRT_iq : Inport  Port=3
  ubiq : Inport  Port=4
  Q_ref : Inport  Port=5
  Divide1 : Product  Inputs=*/
  Gain1 : Gain  Gain=-1
  Gain7 : Gain  Gain=-1
  LVRT Priority : Switch  Threshold=.9  SaturateOnIntegerOverflow=off  InputSameDT=off
  P/Q Priority : Switch  Criteria=u2 ~= 0  SaturateOnIntegerOverflow=off  InputSameDT=off
  PU : Gain  Gain=1/MVA
  Priority Mode : Constant  Value=P-2
  Saturation Dynamic : simulink/Discontinuities/Saturation Dynamic  OutMin=[]  OutMax=[]  OutDataTypeStr=Inherit: Same as second input  OutDataType=fixdt(1, 16)  OutScaling=2^-10  DoSatur=off
  Saturation2 : Saturate  UpperLimit=1  LowerLimit=-1
  Saturation3 : Saturate  UpperLimit=Imax  LowerLimit=-Imax
  Sum : Sum  Inputs=|++
  Sum1 : Sum  Inputs=|-+
  droop m_v : Gain  Gain=mv
  ubiq1 : InportShadow  Port=4
  iq_ref : Outport
  wires:
  LVRT Priority/1 -> iq_ref/1
  Sum1/1 -> droop m_v/1
  P/Q Priority/1 -> LVRT Priority/1
  Gain1/1 -> LVRT Priority/3
  ubiq/1 -> Saturation Dynamic/1
  Saturation2/1 -> Gain1/1
  Saturation3/1 -> P/Q Priority/3
  Priority Mode/1 -> P/Q Priority/2
  Divide1/1 -> Saturation Dynamic/2, Saturation3/1
  Saturation Dynamic/1 -> P/Q Priority/1
  Gain7/1 -> Saturation Dynamic/3
  V_ref/1 -> Sum1/1
  LVRT_iq/1 -> Saturation2/1
  V_mag/1 -> Sum1/2, LVRT Priority/2, Divide1/2
  ubiq1/1 -> Gain7/1
  droop m_v/1 -> Sum/2
  Sum/1 -> Divide1/1
  Q_ref/1 -> PU/1
  PU/1 -> Sum/1

== system TestonBESSPVPlant/BESS PV PARK/60 MWhr Battery Energy Storage/Variant Subsystem/Grid Forming VSM/GridFormingController/Current Limiting/CurrentLimitingMethod ==
  Igd : Inport
  Igq : Inport  Port=2
  currentLimitAndVirtual : Subsystem  VariantControl=both
  currentSaturation : Subsystem  VariantControl=ctSat
  virtualImpedance : Subsystem  VariantControl=virimp
  delVd : Outport
  delVq : Outport  Port=2
  Idmax : Outport  Port=3
  Iqmax : Outport  Port=4

== system TestonBESSPVPlant/BESS PV PARK/60 MWhr Battery Energy Storage/Variant Subsystem/Grid Forming VSM/GridFormingController/Grid Voltage Reactive Power Support/Modifying Active Power Reference ==
  PrefInput : Inport
  Vd : Inport  Port=2
  Igd : Inport  Port=3
  Igq : Inport  Port=4
  AND : Logic  IconShape=distinctive  AllPortsSameDT=off  OutDataTypeStr=boolean
  Abs : Abs  SaturateOnIntegerOverflow=off
  Compare To Constant : simulink/Logic and Bit Operations/Compare To Constant  relop=<=  const=0.90  OutDataTypeStr=boolean
  Computing New Active Power Ref : Subsystem
  Math Function1 : Math  Operator=hypot
  Power Sign : Signum
  Product : Product
  Relay : Relay  OnSwitchValue=maxVICurrentLimit*0.96  OffSwitchValue=1
  Switch : Switch  Criteria=u2 > Threshold  SaturateOnIntegerOverflow=off  InputSameDT=off
  Pref : Outport
  wires:
  Computing New Active Power Ref/1(Pref) -> Switch/1
  Math Function1/1 -> Relay/1  "Is"
  Vd/1 -> Computing New Active Power Ref/2(Vd), Compare To Constant/1
  PrefInput/1 -> Power Sign/1, Switch/3
  Igd/1 -> Math Function1/2
  Igq/1 -> Computing New Active Power Ref/1(Iq), Math Function1/1
  Switch/1 -> Abs/1
  Abs/1 -> Product/1
  Power Sign/1 -> Product/2
  Product/1 -> Pref/1
  Relay/1 -> AND/2
  AND/1 -> Switch/2
  Compare To Constant/1 -> AND/1

== system TestonBESSPVPlant/BESS PV PARK/60 MWhr Battery Energy Storage/Variant Subsystem/Grid Forming VSM/GridFormingController/Grid Voltage Reactive Power Support/Modifying Reactive Power Reference ==
  Vgd : Inport
  Vgq : Inport  Port=2
  Qref : Inport  Port=3
  Pref : Inport  Port=4
  Changing the Power Reference : Subsystem
  Hysteresis : Subsystem
  Math Function : Math  Operator=hypot
  Merge : Merge
  Merge1 : Merge
  NOT : Logic  Operator=NOT  IconShape=distinctive  AllPortsSameDT=off  OutDataTypeStr=boolean
  Not Altering the Power Reference : Subsystem
  PrefNew : Outport
  QrefNew : Outport  Port=2
  wires:
  Vgd/1 -> [Vd], Math Function/1
  Math Function/1 -> Hysteresis/1(Vs), [Vs]
  [Vs] -> Changing the Power Reference/1(Vs)
  Not Altering the Power Reference/1(Prefv) -> Merge/2
  Changing the Power Reference/1(Prefv) -> Merge/1
  NOT/1 -> Not Altering the Power Reference/Enable
  Qref/1 -> Not Altering the Power Reference/2(Qref), [Qref]
  Hysteresis/1(LVFlag) -> Changing the Power Reference/Enable, NOT/1
  [Vd] -> Changing the Power Reference/2(Vd)
  Vgq/1 -> Math Function/2
  Pref/1 -> Not Altering the Power Reference/1(Pref), [Pref]
  Merge1/1 -> QrefNew/1
  Merge/1 -> PrefNew/1
  [Pref] -> Changing the Power Reference/3(Pref)
  [Qref] -> Changing the Power Reference/4(Qref)
  Not Altering the Power Reference/2(Qrefv) -> Merge1/2
  Changing the Power Reference/2(Qrefv) -> Merge1/1

== system TestonBESSPVPlant/BESS PV PARK/60 MWhr Battery Energy Storage/Variant Subsystem/Grid Forming VSM/GridFormingController/Measurement/Frequency Measurement ==
  Vabc : Inport
  Convert To PU : Gain  Gain=1/powerFreq
  Frequency Measurement : Subsystem  TreatAsAtomicUnit=on  SystemSampleTime=sampleTime  mask{initialFrequency=powerFreq, sampleTime=activePowerSampleTime}
      mask prompts: initialFrequency "Initial frequency in Hz"; sampleTime "Sample time in sec"
      mask DialogControl Container7 Prompt: General
  Low-Pass Filter : eeGeneralControl/Low-Pass Filter (Discrete or Continuous)  K=1  T=freqMeasTimeConst  B=inf  A=-inf  init_option=Inherited from block input  x0=0  Ts=-1
  freq : Outport
  wires:
  Low-Pass Filter/1 -> Convert To PU/1  "Freq"
  Frequency Measurement/1(Freq) -> Low-Pass Filter/1
  Convert To PU/1 -> freq/1
  Vabc/1 -> Frequency Measurement/1(abc)

== system TestonBESSPVPlant/BESS PV PARK/60 MWhr Battery Energy Storage/Variant Subsystem/Grid Forming VSM/GridFormingController/Measurement/abc2dq ==
  Igabc : Inport
  Angle : Inport  Port=2
  Vgabc : Inport  Port=3
  Supply Current to dq : Subsystem
  Supply Voltage  to dq : Subsystem
  Vgd : Outport
  Vgq : Outport  Port=2
  Igd : Outport  Port=3
  Igq : Outport  Port=4
  wires:
  Angle/1 -> Supply Voltage  to dq/1(Angle), Supply Current to dq/2(Angle)
  Vgabc/1 -> Supply Voltage  to dq/2(abc)
  Igabc/1 -> Supply Current to dq/1(abc)
  Supply Current to dq/1(Igd) -> Igd/1  "Id"
  Supply Current to dq/2(Igq) -> Igq/1  "Iq"
  Supply Voltage  to dq/1(Vgd) -> Vgd/1  "Vgd"
  Supply Voltage  to dq/2(Vgq) -> Vgq/1  "Vgq"

== system TestonBESSPVPlant/BESS PV PARK/60 MWhr Battery Energy Storage/Variant Subsystem/Grid Forming VSM/GridFormingController/Power Control/ActivePowerControl ==
  Pref : Inport
  Pmeas : Inport  Port=2
  fgrid : Inport  Port=3
  droopControl : Subsystem  VariantControl=droop
  vsmControl : Subsystem  VariantControl=vsm
  Theta : Outport
  w : Outport  Port=2

== system TestonBESSPVPlant/BESS PV PARK/60 MWhr Battery Energy Storage/Variant Subsystem/Grid Forming VSM/GridFormingController/Power Control/ReactiveControl ==
  note: Vs-delV
  Qref : Inport
  Qmeas : Inport  Port=2
  Constant : Constant  Value=voltreference
  Constant2 : Constant  Value=0
  Gain : Gain  Gain=QVoltDroop
  Low-Pass Filter (Discrete or Continuous) : eeGeneralControl/Low-Pass Filter (Discrete or Continuous)  K=1  T=QVoltFilterTC  B=inf  A=-inf  init_option=Specify as parameter  x0=0  Ts=activePowerSampleTime
  Rate Transition : RateTransition
  Rate Transition1 : RateTransition
  Saturation1 : Saturate  UpperLimit=(dcBusVoltage/2)/(sqrt(2/3)*girdLineVoltage)  LowerLimit=-(dcBusVoltage/2)/(sqrt(2/3)*girdLineVoltage)
  Sum : Sum  Inputs=|+-
  Sum1 : Sum  Inputs=|++
  Vmd : Outport
  Vmq : Outport  Port=2
  wires:
  Sum/1 -> Gain/1
  Qmeas/1 -> Low-Pass Filter (Discrete or Continuous)/1
  Low-Pass Filter (Discrete or Continuous)/1 -> Rate Transition1/1
  Gain/1 -> Sum1/1
  Sum1/1 -> Saturation1/1  "Q"
  Constant/1 -> Sum1/2
  Constant2/1 -> Vmq/1
  Qref/1 -> Rate Transition/1
  Saturation1/1 -> Vmd/1
  Rate Transition/1 -> Sum/1
  Rate Transition1/1 -> Sum/2
